simulink model "Tires"  (R2014a)
settings: Solver=ode45  StartTime=0.0  StopTime=10.0  RelTol=1e-3
model workspace: external: MAT-File Tires.mat (data not in the file)
undefined symbols (not defined in the file or in its folder): At, Bk, Bt, Ck, Ct, Dk, Ek, pt, rb
settings Model: Creator=Nathan  LastModifiedBy=Nathan
settings SolverCC: ZeroCrossControl=DisableAll  ZeroCrossAlgorithm=Adaptive
settings OptimizationCC: InlineParams=on
settings DebuggingCC: UnderspecifiedInitializationDetection=Classic  StateNameClashWarn=warning
settings ModelReferenceCC: ModelReferenceMinAlgLoopOccurrences=on

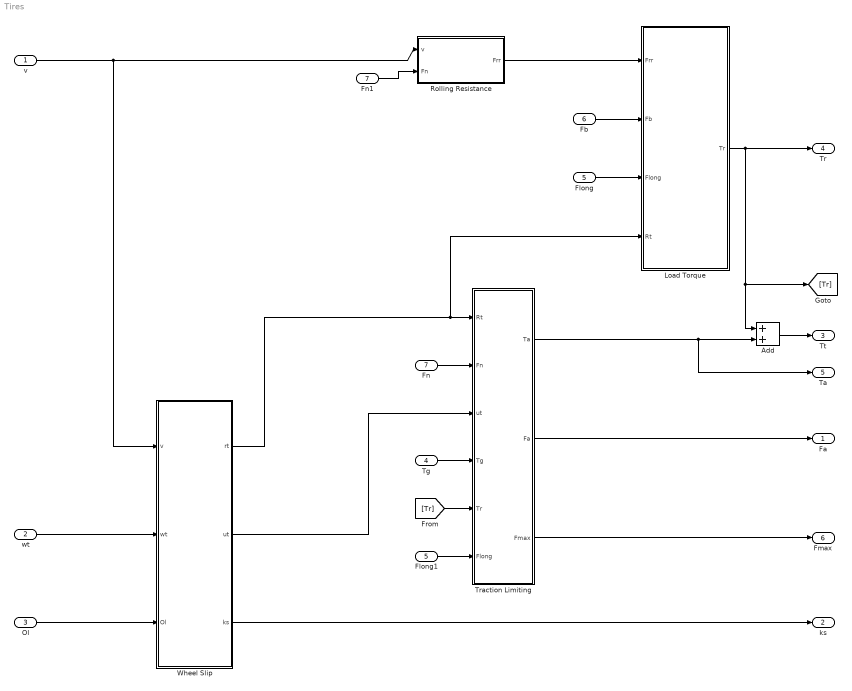
== system Tires ==
  v : Inport
  wt : Inport  Port=2
  Ol : Inport  Port=3
  Tg : Inport  Port=4
  Flong : Inport  Port=5
  Fb : Inport  Port=6
  Fn : Inport  Port=7
  Add : Sum
  Flong1 : InportShadow  Port=5
  Fn1 : InportShadow  Port=7
  Load Torque : Subsystem
  Rolling Resistance : Subsystem
  Traction Limiting : Subsystem
  "Wheel Slip " : Subsystem
  Fa : Outport
  ks : Outport  Port=2
  "Tt " : Outport  Port=3
  Tr : Outport  Port=4
  Ta : Outport  Port=5
  Fmax : Outport  Port=6
  wires:
  v/1 -> "Wheel Slip "/1(v), Rolling Resistance/1(v)
  wt/1 -> "Wheel Slip "/2(wt)
  Ol/1 -> "Wheel Slip "/3(Ol)
  Rolling Resistance/1(Frr) -> Load Torque/1(Frr)
  Tg/1 -> Traction Limiting/4(Tg)
  Fb/1 -> Load Torque/2(Fb)
  Fn/1 -> Traction Limiting/2(Fn)
  "Wheel Slip "/1(rt) -> Load Torque/4(Rt), Traction Limiting/1(Rt)
  Traction Limiting/2(Fa) -> Fa/1
  "Wheel Slip "/3(ks) -> ks/1
  Load Torque/1(Tr) -> Add/1, [Tr], Tr/1
  "Wheel Slip "/2(ut) -> Traction Limiting/3(ut)
  Flong1/1 -> Traction Limiting/6(Flong)
  Flong/1 -> Load Torque/3(Flong)
  [Tr] -> Traction Limiting/5(Tr)
  Add/1 -> "Tt "/1
  Traction Limiting/1(Ta) -> Ta/1, Add/2
  Traction Limiting/3("Fmax ") -> Fmax/1
  Fn1/1 -> Rolling Resistance/2(Fn)

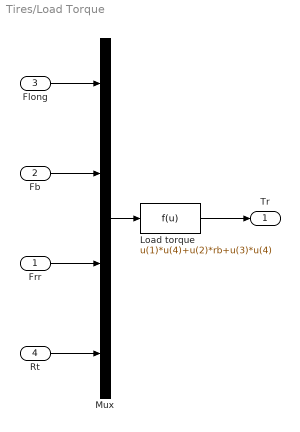
== system Tires/Load Torque ==
  Frr : Inport
  Fb : Inport  Port=2
  Flong : Inport  Port=3
  Rt : Inport  Port=4
  Load torque : Fcn  Expr=u(1)*u(4)+u(2)*rb+u(3)*u(4)
  Mux : Mux
  Tr : Outport
  wires:
  Mux/1 -> Load torque/1
  Load torque/1 -> Tr/1
  Flong/1 -> Mux/1
  Fb/1 -> Mux/2
  Frr/1 -> Mux/3
  Rt/1 -> Mux/4

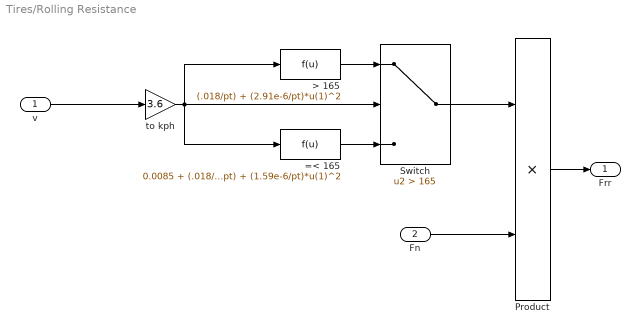
== system Tires/Rolling Resistance ==
  v : Inport
  Fn : Inport  Port=2
  "=< 165 " : Fcn  Expr=0.0085 + (.018/pt) + (1.59e-6/pt)*u(1)^2
  "> 165 " : Fcn  Expr=(.018/pt) + (2.91e-6/pt)*u(1)^2
  Product : Product
  Switch : Switch  Criteria=u2 > Threshold  Threshold=165
  to kph : Gain  Gain=3.6
  Frr : Outport
  wires:
  v/1 -> to kph/1
  to kph/1 -> "=< 165 "/1, "> 165 "/1, Switch/2
  "> 165 "/1 -> Switch/1
  "=< 165 "/1 -> Switch/3
  Switch/1 -> Product/1
  Fn/1 -> Product/2
  Product/1 -> Frr/1

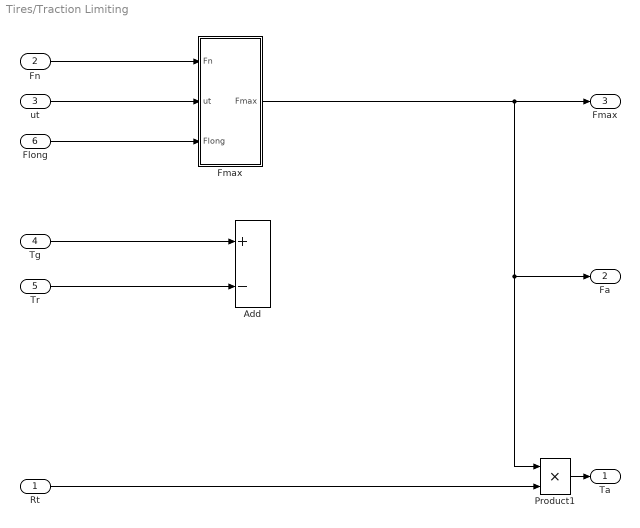
== system Tires/Traction Limiting ==
  Rt : Inport
  Fn : Inport  Port=2
  ut : Inport  Port=3
  Tg : Inport  Port=4
  Tr : Inport  Port=5
  Flong : Inport  Port=6
  Add : Sum  Inputs=+-
  Fmax : Subsystem
  Product1 : Product
  Ta : Outport
  Fa : Outport  Port=2
  "Fmax " : Outport  Port=3
  wires:
  Tg/1 -> Add/1
  Tr/1 -> Add/2
  Fmax/1(Fmax) -> Fa/1, Product1/1, "Fmax "/1
  Rt/1 -> Product1/2
  Product1/1 -> Ta/1
  Fn/1 -> Fmax/1(Fn)
  ut/1 -> Fmax/2(ut)
  Flong/1 -> Fmax/3(Flong)

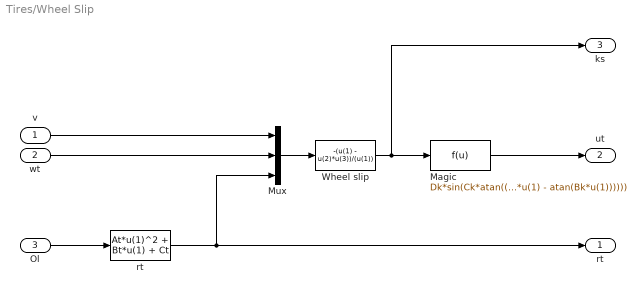
== system Tires/Wheel Slip  ==
  v : Inport
  wt : Inport  Port=2
  Ol : Inport  Port=3
  " rt" : Fcn  Expr=At*u(1)^2 + Bt*u(1) + Ct
  Magic : Fcn  Expr=Dk*sin(Ck*atan(( Bk*u(1) - Ek*(Bk*u(1) - atan(Bk*u(1))))))
  Mux : Mux  Inputs=3
  Wheel slip : Fcn  Expr=-(u(1) - u(2)*u(3))/(u(1))
  rt : Outport
  ut : Outport  Port=2
  ks : Outport  Port=3
  wires:
  Ol/1 -> " rt"/1
  " rt"/1 -> Mux/3, rt/1
  wt/1 -> Mux/2
  Mux/1 -> Wheel slip/1
  v/1 -> Mux/1
  Wheel slip/1 -> ks/1, Magic/1
  Magic/1 -> ut/1

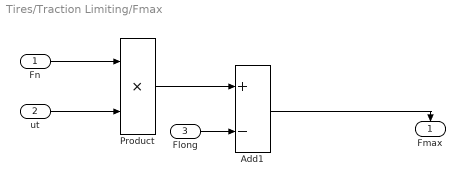
== system Tires/Traction Limiting/Fmax ==
  Fn : Inport
  ut : Inport  Port=2
  Flong : Inport  Port=3
  Add1 : Sum  Inputs=+-
  Product : Product
  Fmax : Outport
  wires:
  ut/1 -> Product/2
  Flong/1 -> Add1/2
  Fn/1 -> Product/1
  Product/1 -> Add1/1
  Add1/1 -> Fmax/1
